simulink model "SIMULACIO_MGD"  (Simulink 7.7)
settings: Solver=ode1  StartTime=0.0  StopTime=inf  RelTol=1e-3
libraries: simulink x4
settings Model: Creator=JohnConstantine  LastModifiedBy=JohnConstantine

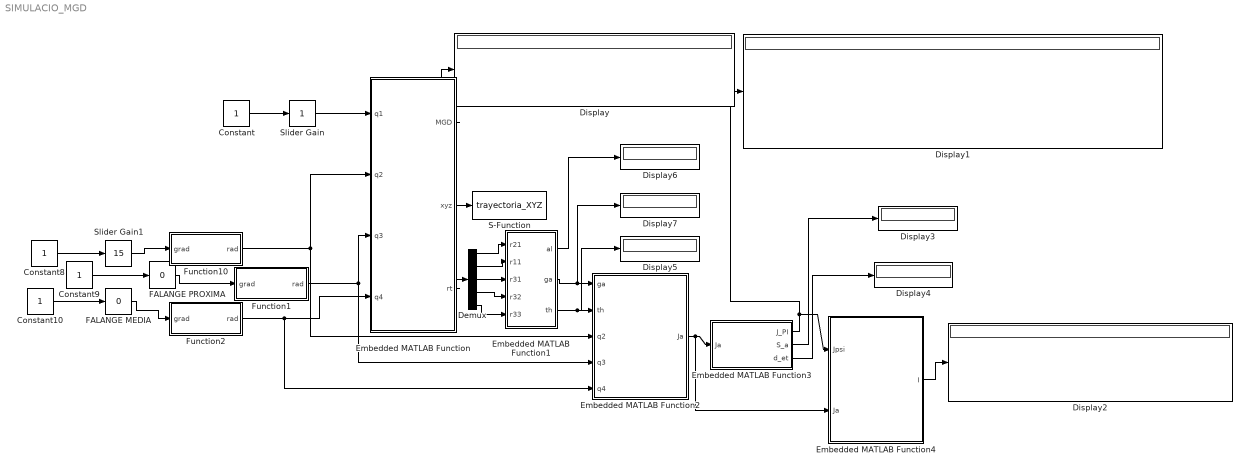
== system SIMULACIO_MGD ==
  Constant{,8..10} (4 alike) : Constant
  Demux : Demux  Outputs=5
  Display{,1..7} (8 alike) : Display
  Embedded MATLAB Function : Stateflow chart  TreatAsAtomicUnit=on
  Embedded MATLAB Function1 : Stateflow chart  TreatAsAtomicUnit=on
  Embedded MATLAB Function2 : Stateflow chart  TreatAsAtomicUnit=on
  Embedded MATLAB Function3 : Stateflow chart  TreatAsAtomicUnit=on
  Embedded MATLAB Function4 : Stateflow chart  TreatAsAtomicUnit=on
  FALANGE MEDIA : simulink/Math Operations/Slider Gain  SystemSampleTime=-1  low=0  gain=0  high=110
  FALANGE PROXIMA : simulink/Math Operations/Slider Gain  SystemSampleTime=-1  low=0  gain=0  high=90
  Function1 : Stateflow chart  TreatAsAtomicUnit=on
  Function10 : Stateflow chart  TreatAsAtomicUnit=on
  Function2 : Stateflow chart  TreatAsAtomicUnit=on
  S-Function : S-Function  FunctionName=trayectoria_XYZ  Parameters=[-10 10 -10 10 -10 10]  EnableBusSupport=off
  Slider Gain : simulink/Math Operations/Slider Gain  SystemSampleTime=-1  low=0  gain=1  high=2.5
  Slider Gain1 : simulink/Math Operations/Slider Gain  SystemSampleTime=-1  low=0  gain=15  high=15
  wires:
  Constant/1 -> Slider Gain/1
  Constant8/1 -> Slider Gain1/1
  Constant9/1 -> FALANGE PROXIMA/1
  Constant10/1 -> FALANGE MEDIA/1
  Embedded MATLAB Function/1(MGD) -> Display/1
  Function10/1(rad) -> Embedded MATLAB Function/2(q2), Embedded MATLAB Function2/3(q2)
  Slider Gain1/1 -> Function10/1(grad)
  FALANGE PROXIMA/1 -> Function1/1(grad)
  Function1/1(rad) -> Embedded MATLAB Function/3(q3), Embedded MATLAB Function2/4(q3)
  Function2/1(rad) -> Embedded MATLAB Function2/5(q4), Embedded MATLAB Function/4(q4)
  FALANGE MEDIA/1 -> Function2/1(grad)
  Embedded MATLAB Function/3(rt) -> Demux/1
  Demux/1 -> Embedded MATLAB Function1/1(r21)
  Demux/2 -> Embedded MATLAB Function1/2(r11)
  Demux/3 -> Embedded MATLAB Function1/3(r31)
  Demux/4 -> Embedded MATLAB Function1/4(r32)
  Demux/5 -> Embedded MATLAB Function1/5(r33)
  Embedded MATLAB Function/2(xyz) -> S-Function/1
  Embedded MATLAB Function1/2(ga) -> Embedded MATLAB Function2/1(ga), Display7/1
  Embedded MATLAB Function1/3(th) -> Embedded MATLAB Function2/2(th), Display5/1
  Embedded MATLAB Function2/1(Ja) -> Embedded MATLAB Function3/1(Ja), Embedded MATLAB Function4/2(Ja)
  Embedded MATLAB Function3/1(J_PI) -> Display1/1, Embedded MATLAB Function4/1(Jpsi)
  Embedded MATLAB Function4/1(I) -> Display2/1
  Slider Gain/1 -> Embedded MATLAB Function/1(q1)
  Embedded MATLAB Function3/2(S_a) -> Display3/1
  Embedded MATLAB Function3/3(d_et) -> Display4/1
  Embedded MATLAB Function1/1(al) -> Display6/1

== matlab function Function1 ==
  data: grad input double; rad output double
function rad =grad2rad(grad)

rad=grad*2*pi/360;

== matlab function Embedded MATLAB Function ==
  data: q1 input double; MGD output double; q2 input double; q3 input double; q4 input double; xyz output double; rt output double
function [MGD,xyz,rt] =mgdFalange(q1,q2,q3,q4)

d2=1.20349;
a2=.9907;
a3=.8862;
a4=1.5;
a5=.8862;
a6=1.5;

 MGD=[ -cos(q3 + q4)*sin(q2),  sin(q3 + q4)*sin(q2), cos(q2),                                         -sin(q2)*(a2 + a5*cos(q3 + q4) + a6*cos(q3 + q4) + a3*cos(q3) + a4*cos(q3));...
               -sin(q3 + q4),         -cos(q3 + q4),       0,                                                  - d2 - a5*sin(q3 + q4) - a6*sin(q3 + q4) - a3*sin(q3) - a4*sin(q3);...
        cos(q3 + q4)*cos(q2), -sin(q3 + q4)*cos(q2), sin(q2), q1 + a2*cos(q2) + cos(q2)*cos(q3)*(a3 + a4) - cos(q2)*sin(q3)*sin(q4)*(a5 + a6) + cos(q2)*cos(q3)*cos(q4)*(a5 + a6);...
                           0,                     0,       0,                                                                                                                  1];
                                                                                                                                                                                                                                                                                 
H=MGD;
xyz=[MGD(1,4) MGD(2,4) MGD(3,4)];

% r21=H(2,1);
% r11=H(1,1);
% r31=H(3,1);
% r32=H(3,2);
% r33=H(3,3);



rt=[H(2,1) H(1,1) H(3,1) H(3,2) H(3,3);];%Las posiciones de la matriz de rotacion de los angulos de EULER y RPY para el calculo de alpha, gamma, theta

== matlab function Function2 ==
  data: grad input double; rad output double
function rad =grad2rad(grad)

rad=grad*2*pi/360;

== matlab function Embedded MATLAB Function1 ==
  data: r21 input double; r11 input double; r31 input double; r32 input double; r33 input double; al output double; ga output double; th output double
function [al,ga,th]=Angulos_Euler(r21,r11,r31,r32,r33)
%rt=[H(2,1) H(1,1) H(3,1) H(3,2) H(3,3);]

%  r21=R(2,1);
%  r11=R(1,1);
%  r31=R(3,1);
%  r32=R(3,2);
%  r33=R(3,3);
  
 th=atan2(r21,r11);%Z
 ga=atan2(-r31,sqrt(r32^2+r33^2)); %Y
 al=atan2(r32,r33);%X

%   Theta=[al ga th].'; % valores de theta

== matlab function Embedded MATLAB Function2 ==
  data: ga input double; th input double; q2 input double; q3 input double; q4 input double; Ja output double
function Ja =Angulos_rotacionales(ga,th,q2,q3,q4)
%rt=[H(2,1) H(1,1) H(3,1) H(3,2) H(3,3);]
d2=1.20349;
a2=.9907;
a3=.8862;
a4=1.5;
a5=.8862;
a6=1.5;


Ja=[ 0, -cos(q2)*(a2 + a5*cos(q3 + q4) + a6*cos(q3 + q4) + a3*cos(q3) + a4*cos(q3)),  sin(q2)*(a5*sin(q3 + q4) + a6*sin(q3 + q4) + a3*sin(q3) + a4*sin(q3)),              sin(q3 + q4)*sin(q2)*(a5 + a6);
     0,                                                                           0,          - a5*cos(q3 + q4) - a6*cos(q3 + q4) - a3*cos(q3) - a4*cos(q3),                     -cos(q3 + q4)*(a5 + a6);
     1, -sin(q2)*(a2 + a5*cos(q3 + q4) + a6*cos(q3 + q4) + a3*cos(q3) + a4*cos(q3)), -cos(q2)*(a5*sin(q3 + q4) + a6*sin(q3 + q4) + a3*sin(q3) + a4*sin(q3)),             -sin(q3 + q4)*cos(q2)*(a5 + a6);
     0,                                                            -sin(th)/cos(ga),                                              (cos(q2)*cos(th))/cos(ga),                   (cos(q2)*cos(th))/cos(ga);
     0,                                                                    -cos(th),                                                       -cos(q2)*sin(th),                            -cos(q2)*sin(th);
     0,                                                            -tan(ga)*sin(th),                            sin(q2) + (cos(q2)*cos(th)*sin(ga))/cos(ga), sin(q2) + (cos(q2)*cos(th)*sin(ga))/cos(ga)];

== matlab function Embedded MATLAB Function3 ==
  data: Ja input double; J_PI output double; S_a output double; d_et output double
function [J_PI,S_a,d_et]  = Angulos_rotacionales(Ja)

Sa=Ja.'*Ja;
 lambda=0.01;
 %J_ainv=(Ja.'*Ja)\Ja.';
 
 %J_ainv=(Ja.'*Ja + lambda*eye(4))\Ja.';
S_a=Sa(4,4);
 if (Sa(4,4) < lambda )
     J_PI=(Ja.'*Ja + lambda*eye(4))\Ja.';
 else 
     %%J_ainv=(Ja.'*Ja)\Ja.';
       J_PI= pinv(Ja);
 end
 
 d_et= det(Sa);

%J_PI=(Ja.'*Ja)\Ja.'; %el punto es para que me de el resultado real de la transpuesta y no me de la transpuesta conjugada
                     %de este modo "\" se obtiene la inversa de la matriz y al mismo tiempo multiplico por JaT

%J_PI=(Ja.'*Ja+lambda*eye(4))\Ja.';
%%J_PI_2=pinv(Ja); Comando "pinv" de MATLAB para obtener la PSEUDOINVERSA

== matlab function Embedded MATLAB Function4 ==
  data: Jpsi input double; Ja input double; I output double
function I =Angulos_rotacionales(Jpsi,Ja)
%rt=[H(2,1) H(1,1) H(3,1) H(3,2) H(3,3);]
I=Jpsi*Ja;

== matlab function Function10 ==
  data: grad input double; rad output double
function rad =grad2rad(grad)

rad=grad*2*pi/360;
